simulink model "MassSpringODE"  (R2022a)
settings: Solver=VariableStepAuto  StartTime=0.0  StopTime=50  RelTol=1e-3
undefined symbols (not defined in the file): b, k, m
settings Model: Creator=Adam Ghatta  LastModifiedBy=Adam Ghatta

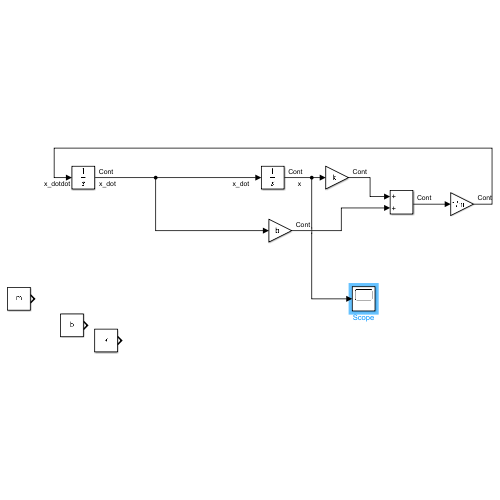
[thumbnail: Simulink's stored preview of the top-level diagram]
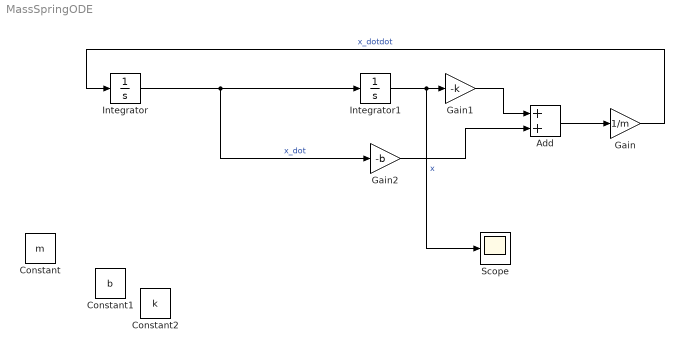
== system MassSpringODE ==
  Add : Sum
  Constant : Constant  Value=m
  Constant1 : Constant  Value=b
  Constant2 : Constant  Value=k
  Gain : Gain  Gain=1/m
  Gain1 : Gain  Gain=-k
  Gain2 : Gain  Gain=-b
  Integrator : Integrator
  Integrator1 : Integrator  InitialCondition=5
  Scope : Scope
  wires:
  Integrator/1 -> Gain2/1, Integrator1/1  "x_dot"
  Gain/1 -> Integrator/1  "x_dotdot"
  Integrator1/1 -> Scope/1, Gain1/1  "x"
  Gain1/1 -> Add/1
  Gain2/1 -> Add/2
  Add/1 -> Gain/1
